simulink model "Cularis_server_vortextest"  (Simulink 8.6)
settings: Solver=FixedStepAuto  SolverMode=SingleTasking  StartTime=0.0  StopTime=uavsim.simConfig.tsim  FixedStep=uavsim.simConfig.tsample_model  RelTol=1
model workspace (MAT data in the model file):
  VortexSig = Simulink.Signal
  VortexSig.DataType = 'Bus: VortexStates'
  VortexSig.Units = 'auto'
  VortexSig.Dimensions = [10 1]
  VortexSig.DimensionsMode = 'Fixed'
  VortexSig.Complexity = 'real'
  VortexSig.SampleTime = -1
  VortexSig.SamplingMode = 'auto'
  VortexSig.InitialValue = 'VortexStates_MATLABStruct_array'
undefined symbols (not defined in the file or in its folder): DiscIntNeverNeededParam, uavsim
libraries: aerolibtransform2 x7, aerolibutil x3, uavsimBlockset_UAV3DInterface x3, uavsimblockset x2, simulink_extras x1, uavsimBlockset_Cularis_withUAV3D x1, aerolibanimutils x1
settings Model: Creator=mstolle  LastModifiedBy=j.bolting  ExtModeTrigDuration=100
settings SolverCC: ZcThreshold=1e-5  ZeroCrossAlgorithm=Adaptive  AlgebraicLoopSolver=LineSearch  AutoInsertRateTranBlk=on
settings DataIOCC: LimitDataPoints=off  SaveFinalState=on  SaveFormat=StructureWithTime  SignalLoggingSaveFormat=Dataset  SaveOutput=off  SaveState=on  DSMLogging=off  InspectSignalLogs=on  StateSaveName=tmp_raccel_xout
settings OptimizationCC: BlockReduction=off  OptimizeBlockIOStorage=off  BufferReuse=off  GlobalBufferReuse=off  ExpressionFolding=off  LocalBlockOutputs=off  EfficientMapNaN2IntZero=off  SimCompilerOptimization=on
settings DebuggingCC: UnderspecifiedInitializationDetection=Simplified  MergeDetectMultiDrivingBlocksExec=error  IgnoredZcDiagnostic=none  FcnCallInpInsideContextMsg=EnableAllAsError  BusObjectLabelMismatch=error
settings HardwareCC: TargetBitPerPointer=64  TargetLongLongMode=on  TargetIntDivRoundTo=Zero  TargetEndianess=LittleEndian  TargetWordSize=64  TargetHWDeviceType=MATLAB Host  ProdEqTarget=off
settings ModelReferenceCC: UpdateModelReferenceTargets=IfOutOfDate  ModelReferenceNumInstancesAllowed=Single  ModelReferenceMinAlgLoopOccurrences=on
settings SFSimCC: SFSimEcho=off
settings RTWCC: SystemTargetFile=raccel.tlc  TemplateMakefile=raccel_default_tmf  RTWVerbose=off  RTWUseSimCustomCode=on
settings CodeAppCC: GenerateComments=off  MaxIdLength=128  SimulinkBlockComments=off
settings RaccelTargetCC: ERTMultiwordTypeDef=System defined  ERTMultiwordLength=256  GeneratePreprocessorConditionals=Use local settings  ERTFirstTimeCompliant=off  MultiInstanceERTCode=off  ENABLE_SLEXEC_SSBRIDGE=0  RTWCAPIParams=on
settings ConfigComp: CovSFcnEnable=off
settings ConfigurationSet: Description=SimMechanics 2G

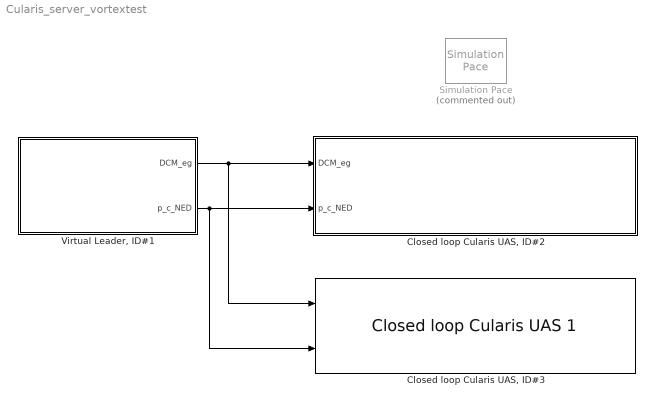
== system Cularis_server_vortextest ==
  "Closed loop Cularis UAS, ID#2" : Subsystem  AncestorBlock=uavsimblockset/Closed loop Cularis UAS 1  mask{closedloopmask_ID=2}
      mask prompts: closedloopmask_ID "UAS ID"
  "Closed loop Cularis UAS, ID#3" : uavsimblockset/Closed loop Cularis UAS 1  closedloopmask_ID=3
  Simulation Pace : aerolibanimutils/Simulation Pace  Commented=on  SimulationPace=1  SleepMode=MATLAB Thread  OutputPaceError=off  SampleTime=-1
  "Virtual Leader, ID#1" : Subsystem  mask{aircraftmask_phithetapsi0=uavsim.formation(1).phithetapsi0, aircraftmask_p0_NED_m=uavsim.formation(1).p0_NED', aircraftmask_originNED_ECEF_rrm=uavsim.originNED_ECEF_radradm, aircraftmask_pqr0=uavsim.formation(1).omega0, aircraftmask_uvw0=uavsim.formation(1).uvw0, aircraftmask_phithetapsi_trim=uavsim.formation(1).phithetapsi0, aircraftmask_ID=1, aircraftmask_wakevortexenabled=on, aircraftmask_navigationLaw=-1, uavsim=uavsim, leaderID=0, airkraftmask_displayLeader=on}
      mask prompts: aircraftmask_phithetapsi0 "Initial Euler angles [rad]"; aircraftmask_p0_NED_m "Initial position, NED frame [m]"; aircraftmask_originNED_ECEF_rrm "Origin NED frame. ECEF, [rad rad m]"; aircraftmask_pqr0 "Initial rotation rates, body frame [rad/s]"; aircraftmask_uvw0 "Initial velocity, body frame [m/s]"; aircraftmask_phithetapsi_trim "Trim Euler angles [rad]"; aircraftmask_ID "Aircraft ID"; aircraftmask_wakevortexenabled "Wake vortex interaction enabled"; aircraftmask_navigationLaw "Active navigation law (-1: automatic selection)"; uavsim "Parameter set"; leaderID "Follows which ID?"; airkraftmask_displayLeader "Display virtual leader"
      mask Display:
      | % Set Icon:
      | %image(imread('images/cularis.png'), [.2, .2, .6, .6])
  wires:
  "Virtual Leader, ID#1"/1(DCM_eg) -> "Closed loop Cularis UAS, ID#2"/1(DCM_eg), "Closed loop Cularis UAS, ID#3"/1
  "Virtual Leader, ID#1"/2(p_c_NED) -> "Closed loop Cularis UAS, ID#2"/2(p_c_NED), "Closed loop Cularis UAS, ID#3"/2

== system Cularis_server_vortextest/Closed loop Cularis UAS, ID#2 ==
  DCM_eg : Inport
  p_c_NED : Inport  Port=2
  Controllers : Subsystem
  UAV : uavsimBlockset_Cularis_withUAV3D/UAV A  aircraftmask_phithetapsi0=uavsim.formation(closedloopmask_ID).phithetapsi0  aircraftmask_p0_NED_m=uavsim.formation(closedloopmask_ID).p0_NED'  aircraftmask_originNED_ECEF_rrm=uavsim.originNED_ECEF_radradm  aircraftmask_pqr0=uavsim.formation(closedloopmask_ID).omega0  aircraftmask_uvw0=uavsim.formation(closedloopmask_ID).uvw0  aircraftmask_phithetapsi_trim=uavsim.formation(closedloopmask_ID).phithetapsi0  aircraftmask_ID=closedloopmask_ID  aircraftmask_wakevortexenabled=off  aircraftmask_navigationLaw=-1  uavsim=uavsim  leaderID=0  aircraftmask_displayUAV3D=on  aircraftmask_displayVortices=off
  wires:
  UAV/1 -> Controllers/1(AirframeBus)
  UAV/2 -> Controllers/2(id)
  DCM_eg/1 -> Controllers/3(DCM_eg)
  p_c_NED/1 -> Controllers/4(p_c_NED)
  Controllers/1(u) -> UAV/1  "u_c"

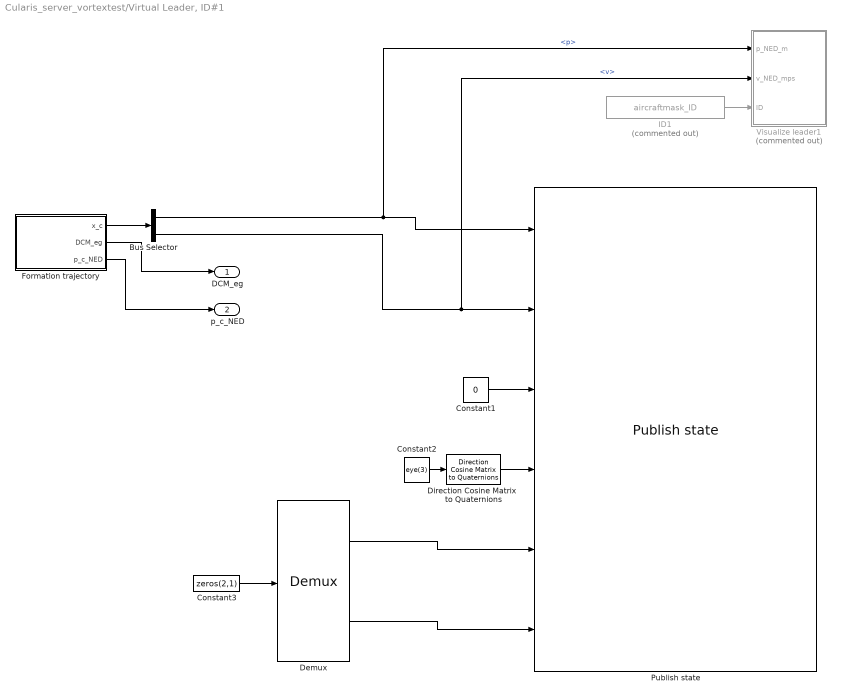
== system Cularis_server_vortextest/Virtual Leader, ID#1 ==
  Bus Selector : BusSelector  OutputSignals=p,v
  Constant1 : Constant  Value=0
  Constant2 : Constant  Value=eye(3)
  Constant3 : Constant  Value=zeros(2,1)
  Demux : Demux  Outputs=2
  Direction Cosine Matrix  to Quaternions : aerolibtransform2/Direction Cosine Matrix  to Quaternions
  Formation trajectory : Subsystem
  ID1 : Constant  Commented=on  Value=aircraftmask_ID
  Publish state : uavsimblockset/Publish state  mask_ID=aircraftmask_ID
  Visualize leader1 : Subsystem  Commented=on  AncestorBlock=formationFlyingBlockset/Visualize leader  TreatAsAtomicUnit=on  SystemSampleTime=uavsim.simConfig.tsample_UAV3D  mask{mask_3dmodel=1}
      mask prompts: mask_3dmodel "3D model"
      mask TypeOptions mask_3dmodel: 0 | 1 | 2 | 3
  DCM_eg : Outport
  p_c_NED : Outport  Port=2
  wires:
  Constant1/1 -> Publish state/3
  Bus Selector/1 -> Publish state/1, Visualize leader1/1(p_NED_m)  "<p>"
  Bus Selector/2 -> Publish state/2, Visualize leader1/2(v_NED_mps)  "<v>"
  Direction Cosine Matrix  to Quaternions/1 -> Publish state/4
  Demux/2 -> Publish state/6
  Demux/1 -> Publish state/5
  Constant2/1 -> Direction Cosine Matrix  to Quaternions/1
  Constant3/1 -> Demux/1
  ID1/1 -> Visualize leader1/3(ID)
  Formation trajectory/1(x_c) -> Bus Selector/1
  Formation trajectory/2(DCM_eg) -> DCM_eg/1
  Formation trajectory/3(p_c_NED) -> p_c_NED/1

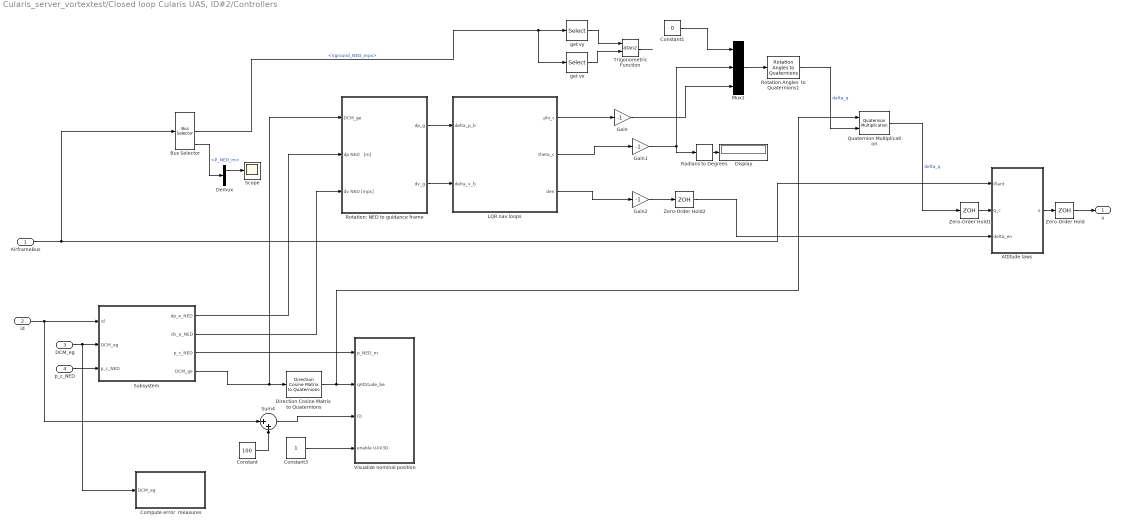
== system Cularis_server_vortextest/Closed loop Cularis UAS, ID#2/Controllers ==
  AirframeBus : Inport
  id : Inport  Port=2
  DCM_eg : Inport  Port=3
  p_c_NED : Inport  Port=4
  Attitude laws : Subsystem  SystemSampleTime=uavsim.ap.hardware.dt_attitudeloops_s
  Bus Selector : BusSelector  OutputSignals=Kinematics.Attitude.DCM_be,Kinematics.Velocity.Vground_NED_mps,Kinematics.Position.P_NED_m
  Compute error  measures : Subsystem
  Constant : Constant  Value=100
  Constant1 : Constant  Value=0
  Constant3 : Constant
  Demux : Demux  Outputs=[2 1]
  Direction Cosine Matrix  to Quaternions : aerolibtransform2/Direction Cosine Matrix  to Quaternions
  Display : Display
  Gain : Gain  Gain=-1
  Gain1 : Gain  Gain=-1
  Gain2 : Gain  Gain=-1
  LQR nav loops : Subsystem  SystemSampleTime=uavsim.ap.hardware.dt_navigationloops_s
  Mux1 : Mux  Inputs=3
  Quaternion Multiplication : aerolibutil/Quaternion Multiplication
  Radians to Degrees : simulink_extras/Transformations/Radians to Degrees
  Rotation Angles  to Quaternions1 : aerolibtransform2/Rotation Angles to Quaternions  rotationOrder=ZYX
  Rotation: NED to guidance frame : Subsystem
  Scope : Scope
  Subsystem : Subsystem
  Sum4 : Sum  Inputs=|++
  Trigonometric Function : Trigonometry  Operator=atan2
  Visualize nominal position : Subsystem  TreatAsAtomicUnit=on  SystemSampleTime=uavsim.simConfig.tsample_UAV3D  mask{mask_3dmodel=1}
      mask prompts: mask_3dmodel "3D model"
      mask TypeOptions mask_3dmodel: 0 | 1 | 2 | 3
  Zero-Order Hold : ZeroOrderHold  SampleTime=uavsim.ap.tsampling_attitudelaws
  Zero-Order Hold1 : ZeroOrderHold  SampleTime=uavsim.ap.tsampling_guidancelaws
  Zero-Order Hold2 : ZeroOrderHold  SampleTime=uavsim.ap.tsampling_guidancelaws
  get vx : Selector  InputPortWidth=3  IndexOptions=Index vector (dialog)  Indices=[1]  OutputSizes=1
  get vy : Selector  InputPortWidth=3  IndexOptions=Index vector (dialog)  Indices=2  OutputSizes=1
  u : Outport
  wires:
  LQR nav loops/3(den) -> Gain2/1
  LQR nav loops/2(theta_c) -> Gain1/1
  LQR nav loops/1(phi_c) -> Gain/1
  Zero-Order Hold/1 -> u/1
  Gain1/1 -> Radians to Degrees/1, Mux1/2
  Trigonometric Function/1 -> ?
  Gain/1 -> Mux1/3
  Mux1/1 -> Rotation Angles  to Quaternions1/1
  get vx/1 -> Trigonometric Function/2
  AirframeBus/1 -> Attitude laws/1(Plant), Bus Selector/1
  get vy/1 -> Trigonometric Function/1
  Attitude laws/1(u) -> Zero-Order Hold/1
  Quaternion Multiplication/1 -> Zero-Order Hold1/1  "delta_q"
  Rotation: NED to guidance frame/2(dv_g) -> LQR nav loops/2(delta_v_b)
  Gain2/1 -> Zero-Order Hold2/1
  Rotation: NED to guidance frame/1(dp_g) -> LQR nav loops/1(delta_p_b)
  Radians to Degrees/1 -> Display/1
  Bus Selector/2 -> get vx/1, get vy/1  "<Vground_NED_mps>"
  Direction Cosine Matrix  to Quaternions/1 -> Quaternion Multiplication/1, Visualize nominal position/2(qAttitude_be)
  Sum4/1 -> Visualize nominal position/3(ID)
  Constant/1 -> Sum4/2
  Constant3/1 -> Visualize nominal position/4(enable UAV3D)
  Zero-Order Hold1/1 -> Attitude laws/2(q_c)
  Zero-Order Hold2/1 -> Attitude laws/3(delta_en)
  id/1 -> Sum4/1, Subsystem/1(id)
  p_c_NED/1 -> Subsystem/3(p_c_NED)
  Subsystem/3("p_c_NED ") -> Visualize nominal position/1(p_NED_m)
  Subsystem/4(DCM_ge) -> Rotation: NED to guidance frame/1(DCM_ge), Direction Cosine Matrix  to Quaternions/1
  Subsystem/1(dp_e_NED) -> Rotation: NED to guidance frame/2(dp NED   [m])
  Subsystem/2(dv_e_NED) -> Rotation: NED to guidance frame/3(dv NED [mps])
  Bus Selector/3 -> Demux/1  "<P_NED_m>"
  Demux/1 -> Scope/1
  DCM_eg/1 -> Compute error  measures/1(DCM_eg), Subsystem/2(DCM_eg)
  Constant1/1 -> Mux1/1
  Rotation Angles  to Quaternions1/1 -> Quaternion Multiplication/2  "delta_q"

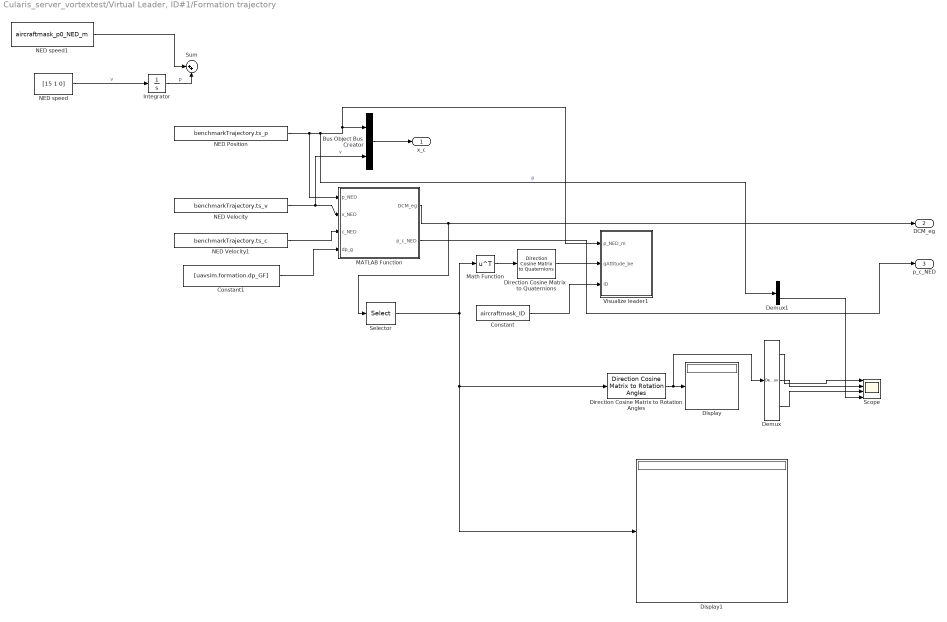
== system Cularis_server_vortextest/Virtual Leader, ID#1/Formation trajectory ==
  Bus Object Bus Creator : BusCreator  Inputs=2  OutDataTypeStr=Bus: svm_bus_x  mask(BUS OBJECT Bus Creator){busType=Bus: svm_bus_x}
      mask prompts: busType "Bus Type"
      mask help:
      | Provides users the cabability to painlessly, instantly customize bus creators of output data type 'Bus:' by selecting the bus object type from a drop down menu dynamically populated by bus objects in the workspace.
      |
      | After pressing the "Apply Selection" button signal lines into the creator are populated and named with the elements in the chosen bus saving the user from having to recall and fill out signal line names.
      |
      | NOTE that when copying a Bus Object Bus Creator from your locked Library the link to the Library is automatically broken. This saves the user from having to Unlock Links To Library (From the Library menu.), Disable Link and finally Break Link (Both from the Model menu.) for every placed instance of the block.
      settings: AttributesFormatString=%<OutDataTypeStr>  CopyFcn=set_param(gcb, 'LinkStatus', 'none')
      mask TypeOptions busType: Bus: AHRS | Bus: Acceleration | Bus: Aero | Bus: Airdata | Bus: Airframe | Bus: Attitude | Bus: CMD | Bus: ControlInfoBus | Bus: Dx | Bus: Enginedata | Bus: Environment | Bus: FlightGearData | Bus: GCSUpstream | Bus: GNSSL1 | Bus: GNSSRTK | Bus: GPS | Bus: IMU | Bus: Kinematics | Bus: LandinggearInput | Bus: MotionTracker | Bus: Position | Bus: Radiodistance | Bus: RotationalAcceleration | Bus: RotationalVelocity | Bus: SensorBus | Bus: StateBus | Bus: Velocity | Bus: VortexParameterBus | Bus: VortexStates | Bus: WindAngles | Bus: iUAScom | Bus: svm_bus_d_exo | Bus: svm_bus_u | Bus: svm_bus_x | Bus: svm_bus_xi
      mask Callback busType:
      | % Using variable names terminated with "_BOBC" to lessen the chances of
      | % collisions with existing workspace variables.
      | 
      | % Get the current block handle and mask handle.
      | handleCreator_BOBC = gcbh;
      | maskObj_BOBC       = Simulink.Mask.get(gcb);
      | 
      | % Get a list of variables in the workspace in order to search for the '1x1
      | % Bus' types.
      | wsVars_BOBC = whos;
      | 
      | % Reset the 'TypeOptions' bus list in case some '1x1 Bus' types have been
      | % deleted from or added to the workspace.
      | maskObj_BOBC.Parameters.TypeOptions = {'<empty>'};
      | 
      | % Reset the bus count.
      | busCount_BOBC = 0;
      | 
      | for index_BOBC = 1:length(wsVars_BOBC)
      | 
      |    % If the variable is a bus object...
      |    if strcmp(wsVars_BOBC(index_BOBC).class, 'Simulink.Bus')
      | 
      |       busCount_BOBC = busCount_BOBC + 1;
      | 
      |       % ... add it to the TypeOptions of the mask.
      |       maskObj_BOBC.Parameters.TypeOptions(busCount_BOBC) = ...
      |                                                            ...
      |                                  {['Bus: ', wsVars_BOBC(index_BOBC).name]};
      |    end
      | end
      | 
      | if busCount_BOBC == 0
      | 
      |    % If there are NO bus objects in the workspace then provide a warning
      |    % popup...
      |    warndlg('There are currently no bus objects in the workspace - you have no use for this block. Use a normal Bus Creator instead.')
      | 
      |    % ... and do nothing.
      | elseif ~strcmp(get_param(handleCreator_BOBC, 'OutDataTypeStr'), 'Inherit: auto')
      | 
      |    % If the currently selected bus data type ('OutDataTypeStr') is not
      |    % 'Inherit: auto' (i.e., if we are reopening the mask.) then get the
      |    % current 'OutDataTypeStr' and 'maskVal.' ('maskVal' is the selected
      |    % 'TypeOptions' list member.)
      |    outDatStr_BOBC = get_param(handleCreator_BOBC, 'OutDataTypeStr');
      |    maskVal_BOBC   = get_param(handleCreator_BOBC, 'MaskValues');
      | 
      |    if ~strcmp(outDatStr_BOBC, maskVal_BOBC{1})
      | 
      |       % Upon re-opening the mask if the default 'TypeOptions' list member
      |       % (The first one.) contained in 'maskVal' does not match the
      |       % currently selected bus data type ('OutDataTypeStr') then set the
      |       % 'TypeOptions' list member to the selected bus data type. (Cuts down
      |       % on confusion to have the displayed list member match the selected
      |       % bus data type rather than the first entry.)
      |       set_param(handleCreator_BOBC, 'MaskValues', {outDatStr_BOBC});
      |    end
      | end
      | 
      | % Clean up the workspace.
      | clear  handleCreator_BOBC  maskObj_BOBC     wsVars_BOBC ...
      |             busCount_BOBC    index_BOBC  outDatStr_BOBC ...
      |              maskVal_BOBC
      mask DialogControl applyMOCBSelection Prompt: Apply Selection
      mask DialogControl applyMOCBSelection Callback:
      | % Using variable names terminated with "_BOBC" to lessen the chances of
      | % collisions with existing workspace variables.
      | 
      | % Get the current block, current block handle and mask handle.
      | currentBlock_BOBC  = gcb;
      | handleCreator_BOBC = gcbh;
      | 
      | % Get the desired bus type...
      | desiredBusType_BOBC = get_param(handleCreator_BOBC, 'busType');
      | 
      | % ... and set the 'OutDataTypeStr' to it.
      | set_param(handleCreator_BOBC, 'OutDataTypeStr', desiredBusType_BOBC);
      | 
      | %% First delete any existing lines on the port.
      | % Get the line handles.
      | lh_BOBC = get_param(handleCreator_BOBC, 'LineHandles');
      | 
      | % If any lines exist (Non- -1 line handles.), delete them and start over.
      | if max(lh_BOBC.Inport > 0)
      | 
      |    for index_BOBC = 1:length(lh_BOBC.Inport)
      | 
      |       if lh_BOBC.Inport(index_BOBC) > 0
      | 
      |          delete_line(lh_BOBC.Inport(index_BOBC))
      |       end
      |    end
      | end
      | 
      | %% Then work on adding new lines.
      | 
      | % Get the block path for 'add_line' function.
      | blockPath_BOBC = get_param(handleCreator_BOBC, 'Parent');
      | 
      | % Get the newly selected bus type ('OutDataTypeStr')...
      | mocbBusType_BOBC = get_param(currentBlock_BOBC, 'OutDataTypeStr');
      | 
      | % ... and parse off "Bus: " so the string of the desired bus contained in
      | % 'OutDataTypeStr' matches the raw workspace bus names.
      | mocbBusType_BOBC = mocbBusType_BOBC(6:end);
      | 
      | % Then evaluate the string containing the workspace bus name which will
      | % load the desired bus parameters.
      | busParams_BOBC = eval(mocbBusType_BOBC);
      | 
      | % From the parameters grab the number of lines to add.
      | numLines_BOBC = length(busParams_BOBC.Elements);
      | 
      | % Set the number of inputs of the masked bus creator to the number of lines
      | % to add.
      | set_param(handleCreator_BOBC, 'Inputs', num2str(numLines_BOBC));
      | 
      | % Get (Inputs.) port handles so we can grab the positions of them.
      | ph_BOBC = get_param(handleCreator_BOBC, 'PortHandles');
      | 
      | for index_BOBC = 1:numLines_BOBC
      | 
      |    % Get the position of input port number 'index_BOBC'.
      |    portPos_BOBC = get_param(ph_BOBC.Inport(index_BOBC), 'Position');
      | 
      |    % Add a line from 50 pixels left of the port position to the port
      |    % position. (This must be done because it's the lines that get named,
      |    % not the port positions.)
      |    portLine_BOBC = add_line(blockPath_BOBC, [portPos_BOBC - [50 0]; portPos_BOBC]);
      | 
      |    % Rename the new line to the bus 'index_BOBC-st/nd/rd/th' element name.
      |    set_param(portLine_BOBC, 'Name', busParams_BOBC.Elements(index_BOBC).Name)
      | end
      | 
      | %% Cleanup the workspace.
      | clear    currentBlock_BOBC  handleCreator_BOBC      index_BOBC ...
      |        desiredBusType_BOBC             lh_BOBC  blockPath_BOBC ...
      |           mocbBusType_BOBC      busParams_BOBC   numLines_BOBC ...
      |                    ph_BOBC        portPos_BOBC   portLine_BOBC
  Constant : Constant  Value=aircraftmask_ID
  Constant1 : Constant  Value=[uavsim.formation.dp_GF]
  Demux : Demux  Outputs=3
  Demux1 : Demux  Outputs=3
  Direction Cosine Matrix to Rotation Angles : aerolibtransform2/Direction Cosine Matrix to Rotation Angles  rotationOrder=ZYX  lim=Default
      settings: AttributesFormatString=Rotation Order: %<rotationOrder>
  Direction Cosine Matrix  to Quaternions : aerolibtransform2/Direction Cosine Matrix  to Quaternions
  Display : Display
      settings: Decimation=3
  Display1 : Display
      settings: Decimation=3
  Integrator : Integrator  InitialCondition=[0 0 0]
  MATLAB Function : MATLAB Function  TreatAsAtomicUnit=on
  Math Function : Math  Operator=transpose  SaturateOnIntegerOverflow=on
  NED Position : FromWorkspace  VariableName=benchmarkTrajectory.ts_p  SampleTime=0
  NED Velocity : FromWorkspace  VariableName=benchmarkTrajectory.ts_v  SampleTime=0
  NED Velocity1 : FromWorkspace  VariableName=benchmarkTrajectory.ts_c  SampleTime=0
  NED speed : Constant  Value=[15 1 0]
  NED speed1 : Constant  Value=aircraftmask_p0_NED_m
  Scope : Scope  NumInputPorts=4
  Selector : Selector  NumberOfDimensions=3  InputPortWidth=3  IndexOptions=Index vector (dialog),Index vector (dialog),Index vector (dialog)  Indices=1:3,1:3,1  OutputSizes=1,1,1
  Sum : Sum  Inputs=|++
  Visualize leader1 : Subsystem  TreatAsAtomicUnit=on  SystemSampleTime=uavsim.simConfig.tsample_UAV3D  mask{mask_3dmodel=3}
      mask prompts: mask_3dmodel "3D model"
      mask TypeOptions mask_3dmodel: 0 | 1 | 2 | 3
  x_c : Outport  OutDataTypeStr=Bus: svm_bus_x
  DCM_eg : Outport  Port=2
  p_c_NED : Outport  Port=3
  wires:
  NED Position/1 -> MATLAB Function/1(p_NED), Demux1/1, Visualize leader1/1(p_NED_m), Bus Object Bus Creator/1  "p"
  NED speed/1 -> Integrator/1  "v"
  Bus Object Bus Creator/1 -> x_c/1
  Integrator/1 -> Sum/2  "p"
  NED speed1/1 -> Sum/1
  NED Velocity/1 -> MATLAB Function/2(v_NED), Bus Object Bus Creator/2  "v"
  NED Velocity1/1 -> MATLAB Function/3(c_NED)
  Selector/1 -> Display1/1, Direction Cosine Matrix to Rotation Angles/1, Math Function/1
  Direction Cosine Matrix  to Quaternions/1 -> Visualize leader1/2(qAttitude_be)
  Constant/1 -> Visualize leader1/3(ID)
  Direction Cosine Matrix to Rotation Angles/1 -> Demux/1, Display/1
  Demux/2 -> Scope/2
  Demux/3 -> Scope/3
  Demux/1 -> Scope/1
  Demux1/3 -> Scope/4
  Constant1/1 -> MATLAB Function/4(dp_g)
  MATLAB Function/1(DCM_eg) -> Selector/1, DCM_eg/1
  MATLAB Function/2(p_c_NED) -> p_c_NED/1
  Math Function/1 -> Direction Cosine Matrix  to Quaternions/1

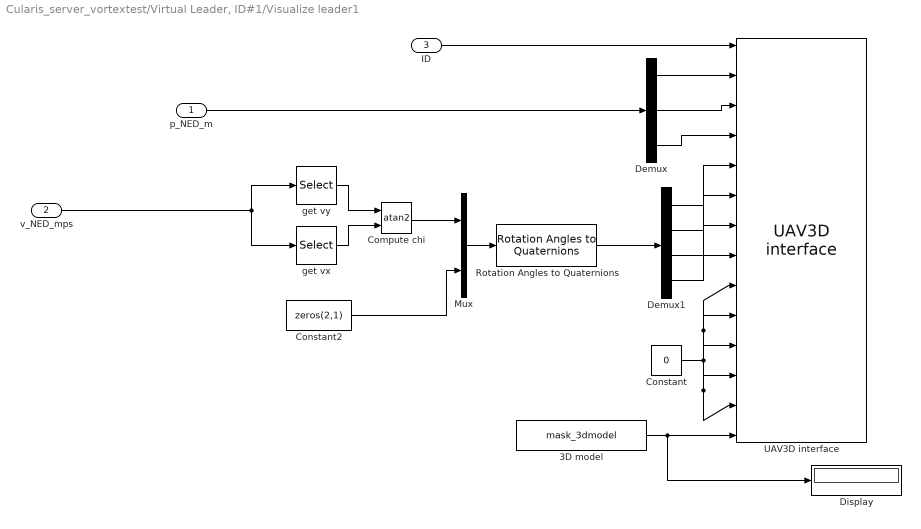
== system Cularis_server_vortextest/Virtual Leader, ID#1/Visualize leader1 ==
  p_NED_m : Inport
  v_NED_mps : Inport  Port=2
  ID : Inport  Port=3
  3D model : Constant  Value=mask_3dmodel
  Compute chi : Trigonometry  Operator=atan2
  Constant : Constant  Value=0
  Constant2 : Constant  Value=zeros(2,1)
  Demux : Demux  Outputs=3
  Demux1 : Demux
  Display : Display
  Mux : Mux  Inputs=2
  Rotation Angles to Quaternions : aerolibtransform2/Rotation Angles to Quaternions  rotationOrder=ZYX
  UAV3D interface : uavsimBlockset_UAV3DInterface/UAV3D interface  ip='localhost'  udpport=4445
  get vx : Selector  InputPortWidth=3  IndexOptions=Index vector (dialog)  Indices=1  OutputSizes=1
  get vy : Selector  InputPortWidth=3  IndexOptions=Index vector (dialog)  Indices=2  OutputSizes=1
  wires:
  Demux/1 -> UAV3D interface/2
  Demux/2 -> UAV3D interface/3
  Demux/3 -> UAV3D interface/4
  Demux1/1 -> UAV3D interface/5
  Demux1/2 -> UAV3D interface/6
  Demux1/4 -> UAV3D interface/8
  get vy/1 -> Compute chi/1
  get vx/1 -> Compute chi/2
  Constant2/1 -> Mux/2
  Mux/1 -> Rotation Angles to Quaternions/1
  Rotation Angles to Quaternions/1 -> Demux1/1
  Compute chi/1 -> Mux/1
  Demux1/3 -> UAV3D interface/7
  Constant/1 -> UAV3D interface/13, UAV3D interface/12, UAV3D interface/11, UAV3D interface/10, UAV3D interface/9
  3D model/1 -> Display/1, UAV3D interface/14
  ID/1 -> UAV3D interface/1
  p_NED_m/1 -> Demux/1
  v_NED_mps/1 -> get vy/1, get vx/1

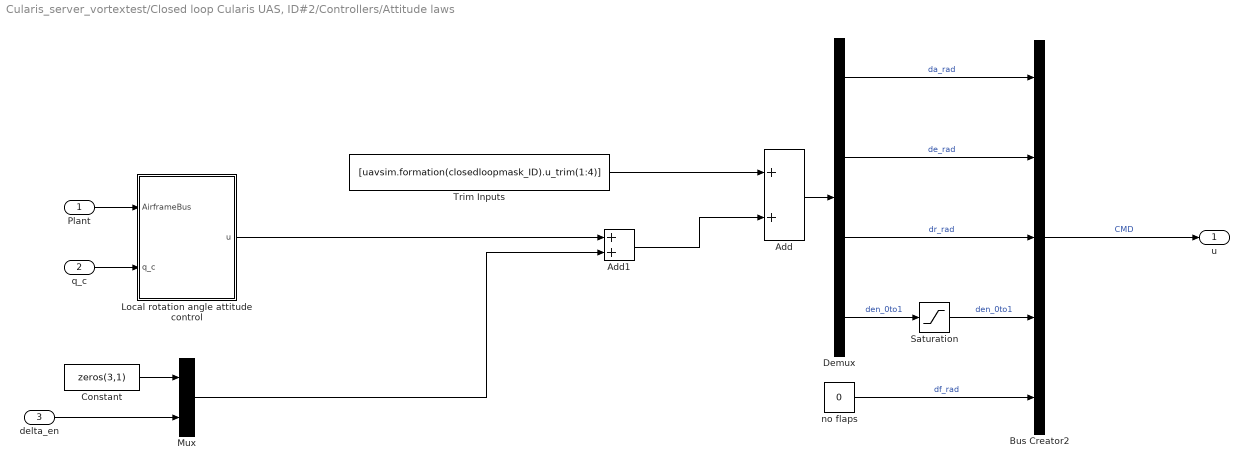
== system Cularis_server_vortextest/Closed loop Cularis UAS, ID#2/Controllers/Attitude laws ==
  Plant : Inport  OutDataTypeStr=Bus: Airframe
  q_c : Inport  Port=2
  delta_en : Inport  Port=3
  Add : Sum
  Add1 : Sum
  Bus Creator2 : BusCreator  Inputs=5  OutDataTypeStr=Bus: CMD  NonVirtualBus=on
  Constant : Constant  Value=zeros(3,1)
  Demux : Demux
  Local rotation angle attitude  control : Subsystem
  Mux : Mux  Inputs=2
  Saturation : Saturate  UpperLimit=1  LowerLimit=0
  Trim Inputs : Constant  Value=[uavsim.formation(closedloopmask_ID).u_trim(1:4)]
  no flaps : Constant  Value=0
  u : Outport  OutDataTypeStr=Bus: CMD
  wires:
  no flaps/1 -> Bus Creator2/5  "df_rad"
  delta_en/1 -> Mux/2
  Add1/1 -> Add/2
  Mux/1 -> Add1/2
  Constant/1 -> Mux/1
  q_c/1 -> Local rotation angle attitude  control/2(q_c)
  Plant/1 -> Local rotation angle attitude  control/1(AirframeBus)
  Add/1 -> Demux/1
  Trim Inputs/1 -> Add/1
  Demux/2 -> Bus Creator2/2  "de_rad"
  Demux/1 -> Bus Creator2/1  "da_rad"
  Saturation/1 -> Bus Creator2/4  "den_0to1"
  Demux/3 -> Bus Creator2/3  "dr_rad"
  Bus Creator2/1 -> u/1  "CMD"
  Local rotation angle attitude  control/1(u) -> Add1/1
  Demux/4 -> Saturation/1  "den_0to1"

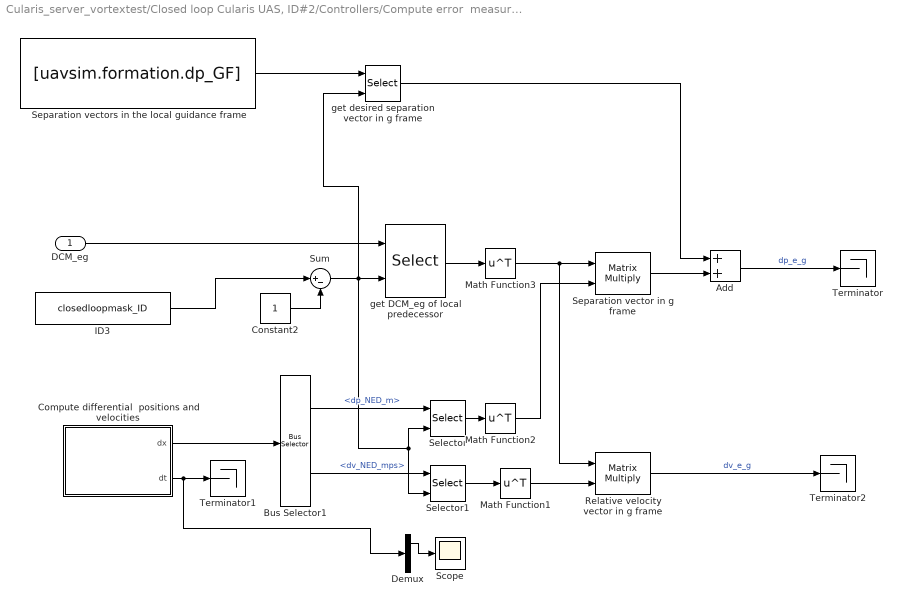
== system Cularis_server_vortextest/Closed loop Cularis UAS, ID#2/Controllers/Compute error  measures ==
  DCM_eg : Inport
  Add : Sum
  Bus Selector1 : BusSelector  OutputSignals=dp_NED_m,dv_NED_mps
  Compute differential  positions and velocities : MATLAB Function  TreatAsAtomicUnit=on
  Constant2 : Constant
  Demux : Demux  Outputs=[4 6]
  ID3 : Constant  Value=closedloopmask_ID
  Math Function1 : Math  Operator=transpose  SaturateOnIntegerOverflow=on
  Math Function2 : Math  Operator=transpose  SaturateOnIntegerOverflow=on
  Math Function3 : Math  Operator=transpose  SaturateOnIntegerOverflow=on
  Relative velocity vector in g frame : Product  Multiplication=Matrix(*)
  Scope : Scope
  Selector : Selector  NumberOfDimensions=2  InputPortWidth=3  IndexOptions=Index vector (port),Select all  Indices=1,1:3  OutputSizes=1,1
  Selector1 : Selector  NumberOfDimensions=2  InputPortWidth=3  IndexOptions=Index vector (port),Index vector (dialog)  Indices=1,1:3  OutputSizes=1,1
  Separation vector in g frame : Product  Multiplication=Matrix(*)
  Separation vectors in the local guidance frame : Constant  Value=[uavsim.formation.dp_GF]
  Sum : Sum  Inputs=|+-
  Terminator : Terminator
  Terminator1 : Terminator
  Terminator2 : Terminator
  get DCM_eg of local predecessor : Selector  NumberOfDimensions=3  InputPortWidth=3  IndexOptions=Index vector (dialog),Index vector (dialog),Index vector (port)  Indices=1:3,1:3,1  OutputSizes=1,1,1
  get desired separation vector in g frame : Selector  NumberOfDimensions=2  InputPortWidth=3  IndexOptions=Select all,Index vector (port)  Indices=1,1:3  OutputSizes=1,1
  wires:
  Separation vectors in the local guidance frame/1 -> get desired separation vector in g frame/1
  DCM_eg/1 -> get DCM_eg of local predecessor/1
  Constant2/1 -> Sum/2
  Bus Selector1/1 -> Selector/1  "<dp_NED_m>"
  Bus Selector1/2 -> Selector1/1  "<dv_NED_mps>"
  Compute differential  positions and velocities/1(dx) -> Bus Selector1/1
  Selector/1 -> Math Function2/1
  ID3/1 -> Sum/1
  Sum/1 -> get desired separation vector in g frame/2, Selector1/2, Selector/2, get DCM_eg of local predecessor/2
  get DCM_eg of local predecessor/1 -> Math Function3/1
  Math Function2/1 -> Separation vector in g frame/2
  Selector1/1 -> Math Function1/1
  Separation vector in g frame/1 -> Add/2
  Add/1 -> Terminator/1  "dp_e_g"
  Relative velocity vector in g frame/1 -> Terminator2/1  "dv_e_g"
  Math Function1/1 -> Relative velocity vector in g frame/2
  Math Function3/1 -> Relative velocity vector in g frame/1, Separation vector in g frame/1
  Compute differential  positions and velocities/2(dt) -> Demux/1, Terminator1/1
  get desired separation vector in g frame/1 -> Add/1
  Demux/1 -> Scope/1

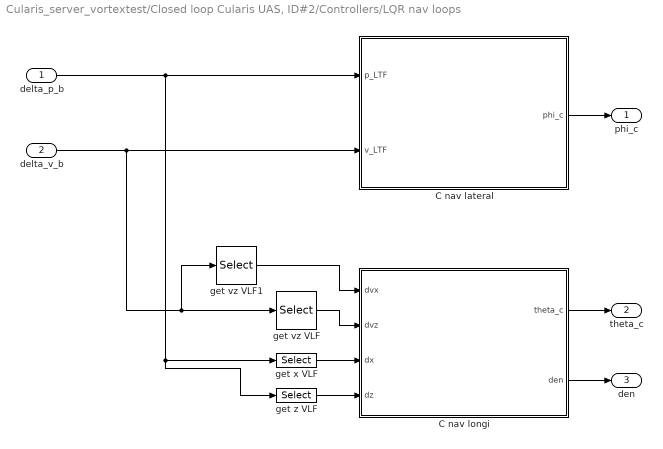
== system Cularis_server_vortextest/Closed loop Cularis UAS, ID#2/Controllers/LQR nav loops ==
  delta_p_b : Inport
  delta_v_b : Inport  Port=2
  C nav lateral : Subsystem
  C nav longi : Subsystem
  get vz VLF : Selector  InputPortWidth=3  IndexOptions=Index vector (dialog)  Indices=3  OutputSizes=1
  get vz VLF1 : Selector  InputPortWidth=3  IndexOptions=Index vector (dialog)  Indices=1  OutputSizes=1
  get x VLF : Selector  InputPortWidth=3  IndexOptions=Index vector (dialog)  Indices=1  OutputSizes=1
  get z VLF : Selector  InputPortWidth=3  IndexOptions=Index vector (dialog)  Indices=3  OutputSizes=1
  phi_c : Outport  PortDimensions=1
  theta_c : Outport  Port=2  PortDimensions=1
  den : Outport  Port=3  PortDimensions=1
  wires:
  C nav longi/2(den) -> den/1
  C nav longi/1(theta_c) -> theta_c/1
  delta_p_b/1 -> C nav lateral/1(p_LTF), get x VLF/1, get z VLF/1
  delta_v_b/1 -> C nav lateral/2(v_LTF), get vz VLF1/1, get vz VLF/1
  C nav lateral/1(phi_c) -> phi_c/1
  get z VLF/1 -> C nav longi/4(dz)
  get x VLF/1 -> C nav longi/3(dx)
  get vz VLF/1 -> C nav longi/2(dvz)
  get vz VLF1/1 -> C nav longi/1(dvx)

== system Cularis_server_vortextest/Closed loop Cularis UAS, ID#2/Controllers/Rotation: NED to guidance frame ==
  DCM_ge : Inport
  dp NED   [m] : Inport  Port=2
  dv NED [mps] : Inport  Port=3
  Rotate position vector from NED to LS frame : Product  Multiplication=Matrix(*)
  Rotate velocity vector from NED to LS frame : Product  Multiplication=Matrix(*)
  dp_g : Outport
  dv_g : Outport  Port=2
  wires:
  Rotate velocity vector from NED to LS frame/1 -> dv_g/1
  Rotate position vector from NED to LS frame/1 -> dp_g/1
  dp NED   [m]/1 -> Rotate position vector from NED to LS frame/2
  dv NED [mps]/1 -> Rotate velocity vector from NED to LS frame/2
  DCM_ge/1 -> Rotate velocity vector from NED to LS frame/1, Rotate position vector from NED to LS frame/1

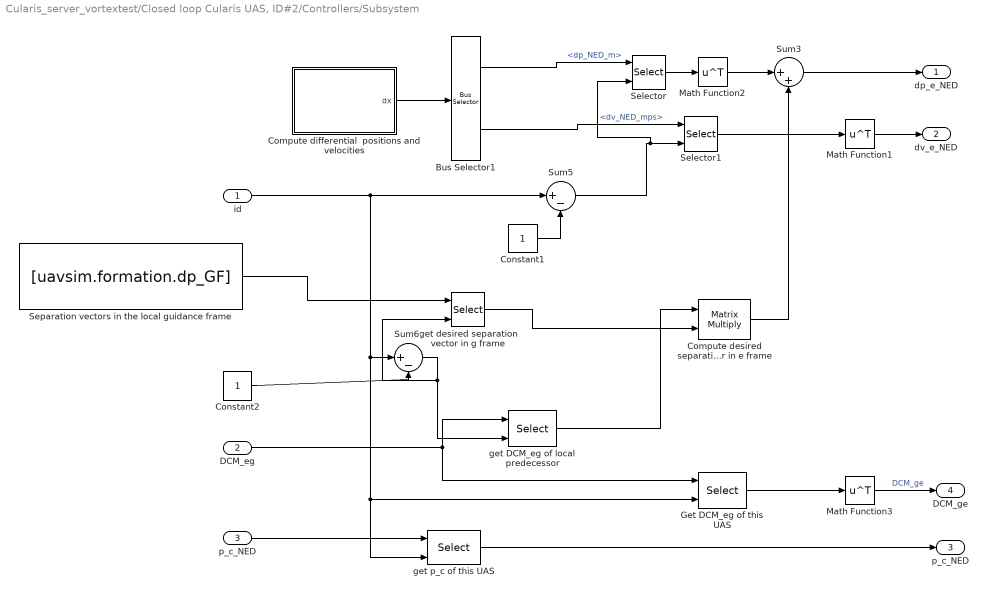
== system Cularis_server_vortextest/Closed loop Cularis UAS, ID#2/Controllers/Subsystem ==
  id : Inport
  DCM_eg : Inport  Port=2
  p_c_NED : Inport  Port=3
  Bus Selector1 : BusSelector  OutputSignals=dp_NED_m,dv_NED_mps
  Compute desired separation vector in e frame : Product  Multiplication=Matrix(*)
  Compute differential  positions and velocities : MATLAB Function  TreatAsAtomicUnit=on
  Constant1 : Constant
  Constant2 : Constant
  Get DCM_eg of this UAS : Selector  NumberOfDimensions=3  InputPortWidth=3  IndexOptions=Index vector (dialog),Index vector (dialog),Index vector (port)  Indices=1:3,1:3,1  OutputSizes=1,1,1
  Math Function1 : Math  Operator=transpose  SaturateOnIntegerOverflow=on
  Math Function2 : Math  Operator=transpose  SaturateOnIntegerOverflow=on
  Math Function3 : Math  Operator=transpose  SaturateOnIntegerOverflow=on
  Selector : Selector  NumberOfDimensions=2  InputPortWidth=3  IndexOptions=Index vector (port),Select all  Indices=1,1:3  OutputSizes=1,1
  Selector1 : Selector  NumberOfDimensions=2  InputPortWidth=3  IndexOptions=Index vector (port),Index vector (dialog)  Indices=1,1:3  OutputSizes=1,1
  Separation vectors in the local guidance frame : Constant  Value=[uavsim.formation.dp_GF]
  Sum3 : Sum  Inputs=|++
  Sum5 : Sum  Inputs=|+-
  Sum6 : Sum  Inputs=|+-
  get DCM_eg of local predecessor : Selector  NumberOfDimensions=3  InputPortWidth=3  IndexOptions=Index vector (dialog),Index vector (dialog),Index vector (port)  Indices=1:3,1:3,1  OutputSizes=1,1,1
  get desired separation vector in g frame : Selector  NumberOfDimensions=2  InputPortWidth=3  IndexOptions=Select all,Index vector (port)  Indices=1,1:3  OutputSizes=1,1
  get p_c of this UAS : Selector  NumberOfDimensions=2  InputPortWidth=3  IndexOptions=Select all,Index vector (port)  Indices=1,1:3  OutputSizes=1,1
  dp_e_NED : Outport
  dv_e_NED : Outport  Port=2
  "p_c_NED " : Outport  Port=3
  DCM_ge : Outport  Port=4
  wires:
  Sum3/1 -> dp_e_NED/1
  Math Function1/1 -> dv_e_NED/1
  p_c_NED/1 -> get p_c of this UAS/1
  get p_c of this UAS/1 -> "p_c_NED "/1
  Constant1/1 -> Sum5/2
  Math Function3/1 -> DCM_ge/1  "DCM_ge"
  Sum5/1 -> Selector/2, Selector1/2
  Compute differential  positions and velocities/1(dx) -> Bus Selector1/1
  Selector1/1 -> Math Function1/1
  Bus Selector1/2 -> Selector1/1  "<dv_NED_mps>"
  Bus Selector1/1 -> Selector/1  "<dp_NED_m>"
  get DCM_eg of local predecessor/1 -> Compute desired separation vector in e frame/1
  Constant2/1 -> Sum6/2
  Sum6/1 -> get DCM_eg of local predecessor/2, get desired separation vector in g frame/2
  Selector/1 -> Math Function2/1
  DCM_eg/1 -> get DCM_eg of local predecessor/1, Get DCM_eg of this UAS/1
  Separation vectors in the local guidance frame/1 -> get desired separation vector in g frame/1
  Get DCM_eg of this UAS/1 -> Math Function3/1
  get desired separation vector in g frame/1 -> Compute desired separation vector in e frame/2
  Math Function2/1 -> Sum3/1
  Compute desired separation vector in e frame/1 -> Sum3/2
  id/1 -> Sum6/1, get p_c of this UAS/2, Get DCM_eg of this UAS/2, Sum5/1

== system Cularis_server_vortextest/Closed loop Cularis UAS, ID#2/Controllers/Visualize nominal position ==
  p_NED_m : Inport
  qAttitude_be : Inport  Port=2
  ID : Inport  Port=3
  enable UAV3D : Inport  Port=4
  3D model : Constant  Value=mask_3dmodel
  Constant : Constant  Value=0
  Demux : Demux  Outputs=3
  Demux1 : Demux
  UAV3D interface : uavsimBlockset_UAV3DInterface/UAV3D interface  ip='localhost'  udpport=4445
  wires:
  Demux/1 -> UAV3D interface/2
  Demux/2 -> UAV3D interface/3
  Demux/3 -> UAV3D interface/4
  Demux1/1 -> UAV3D interface/5
  Demux1/2 -> UAV3D interface/6
  Demux1/4 -> UAV3D interface/8
  qAttitude_be/1 -> Demux1/1
  Demux1/3 -> UAV3D interface/7
  Constant/1 -> UAV3D interface/13, UAV3D interface/12, UAV3D interface/11, UAV3D interface/10, UAV3D interface/9
  3D model/1 -> UAV3D interface/14
  ID/1 -> UAV3D interface/1
  p_NED_m/1 -> Demux/1
  enable UAV3D/1 -> UAV3D interface/Enable

== system Cularis_server_vortextest/Virtual Leader, ID#1/Formation trajectory/Visualize leader1 ==
  p_NED_m : Inport
  qAttitude_be : Inport  Port=2
  ID : Inport  Port=3
  3D model : Constant  Value=mask_3dmodel
  Constant : Constant  Value=0
  Constant1 : Constant
  Demux : Demux  Outputs=3
  Demux1 : Demux
  UAV3D interface : uavsimBlockset_UAV3DInterface/UAV3D interface  ip='localhost'  udpport=4445
  wires:
  Demux/1 -> UAV3D interface/2
  Demux/2 -> UAV3D interface/3
  Demux/3 -> UAV3D interface/4
  Demux1/1 -> UAV3D interface/5
  Demux1/2 -> UAV3D interface/6
  Demux1/4 -> UAV3D interface/8
  qAttitude_be/1 -> Demux1/1
  Demux1/3 -> UAV3D interface/7
  Constant/1 -> UAV3D interface/13, UAV3D interface/12, UAV3D interface/11, UAV3D interface/10, UAV3D interface/9
  3D model/1 -> UAV3D interface/14
  ID/1 -> UAV3D interface/1
  p_NED_m/1 -> Demux/1
  Constant1/1 -> UAV3D interface/Enable

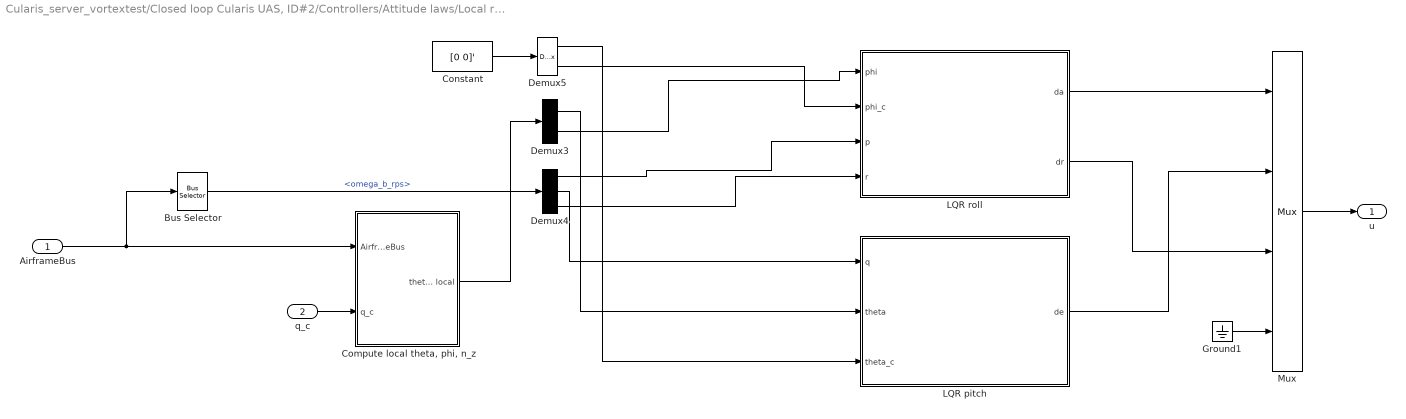
== system Cularis_server_vortextest/Closed loop Cularis UAS, ID#2/Controllers/Attitude laws/Local rotation angle attitude  control ==
  AirframeBus : Inport  OutDataTypeStr=Bus: Airframe
  q_c : Inport  Port=2
  Bus Selector : BusSelector  OutputSignals=Kinematics.RotationalVelocity.omega_b_rps
  "Compute local theta, phi, n_z" : Subsystem
  Constant : Constant  Value=[0 0]'
  Demux3 : Demux  Outputs=2
  Demux4 : Demux  Outputs=3
  Demux5 : Demux  Outputs=2
  Ground1 : Ground
  LQR pitch : Subsystem
  LQR roll : Subsystem
  Mux : Mux
  u : Outport
  wires:
  Ground1/1 -> Mux/4
  AirframeBus/1 -> "Compute local theta, phi, n_z"/1(AirframeBus), Bus Selector/1
  q_c/1 -> "Compute local theta, phi, n_z"/2(q_c)
  Mux/1 -> u/1
  Constant/1 -> Demux5/1
  Bus Selector/1 -> Demux4/1  "<omega_b_rps>"
  "Compute local theta, phi, n_z"/1("theta, phi local") -> Demux3/1
  Demux5/2 -> LQR roll/2(phi_c)
  Demux3/2 -> LQR roll/1(phi)
  Demux4/1 -> LQR roll/3(p)
  Demux4/3 -> LQR roll/4(r)
  Demux5/1 -> LQR pitch/3(theta_c)
  Demux3/1 -> LQR pitch/2(theta)
  Demux4/2 -> LQR pitch/1(q)
  LQR pitch/1(de) -> Mux/2
  LQR roll/1(da) -> Mux/1
  LQR roll/2(dr) -> Mux/3

== system Cularis_server_vortextest/Closed loop Cularis UAS, ID#2/Controllers/LQR nav loops/C nav lateral ==
  p_LTF : Inport
  v_LTF : Inport  Port=2
  Add : Sum  Inputs=+-
  Discrete-Time Integrator1 : DiscreteIntegrator  SampleTime=-1  ICPrevOutput=DiscIntNeverNeededParam  ICPrevScaledInput=DiscIntNeverNeededParam
  Ky : Gain  Gain=uavsim.ap.control.lquadr.latnav.K  Multiplication=Matrix(K*u)
  Mux1 : Mux  Inputs=3
  Selector : Selector  InputPortWidth=3  IndexOptions=Index vector (dialog)  Indices=2  OutputSizes=1
  Selector1 : Selector  InputPortWidth=3  IndexOptions=Index vector (dialog)  Indices=2  OutputSizes=1
  Step : Step  Time=12  After=0
  Trigonometric Function : Trigonometry  Operator=asin
  phi_c : Outport
  wires:
  Ky/1 -> Trigonometric Function/1  "ny_c"
  Selector/1 -> Add/1  "e"
  Step/1 -> Add/2
  Selector1/1 -> Mux1/2
  Discrete-Time Integrator1/1 -> Mux1/3
  Add/1 -> Mux1/1, Discrete-Time Integrator1/1
  Mux1/1 -> Ky/1
  v_LTF/1 -> Selector1/1
  p_LTF/1 -> Selector/1
  Trigonometric Function/1 -> phi_c/1

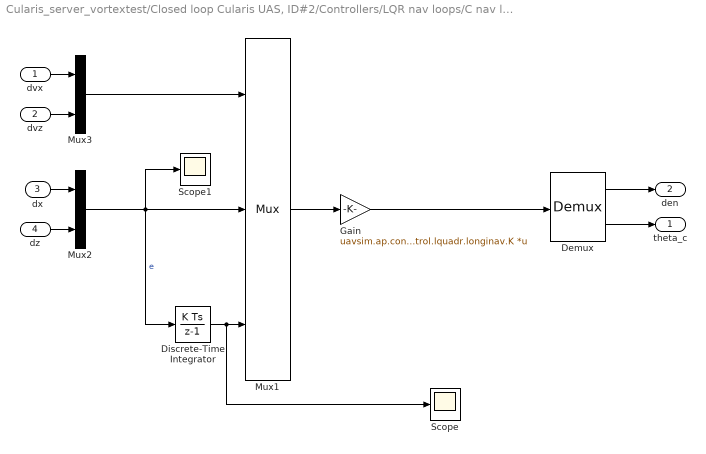
== system Cularis_server_vortextest/Closed loop Cularis UAS, ID#2/Controllers/LQR nav loops/C nav longi ==
  dvx : Inport
  dvz : Inport  Port=2
  dx : Inport  Port=3
  dz : Inport  Port=4
  Demux : Demux  Outputs=2
  Discrete-Time Integrator : DiscreteIntegrator  gainval=1  InitialConditionSetting=State (most efficient)  SampleTime=-1  ICPrevOutput=DiscIntNeverNeededParam  ICPrevScaledInput=DiscIntNeverNeededParam
  Gain : Gain  Gain=uavsim.ap.control.lquadr.longinav.K  Multiplication=Matrix(K*u)
  Mux1 : Mux  Inputs=3
  Mux2 : Mux  Inputs=2
  Mux3 : Mux  Inputs=2
  Scope : Scope
  Scope1 : Scope
  theta_c : Outport
  den : Outport  Port=2
  wires:
  Mux1/1 -> Gain/1
  Demux/1 -> den/1
  Demux/2 -> theta_c/1
  dx/1 -> Mux2/1
  dvz/1 -> Mux3/2
  dvx/1 -> Mux3/1
  Discrete-Time Integrator/1 -> Scope/1, Mux1/3
  Mux2/1 -> Discrete-Time Integrator/1, Scope1/1, Mux1/2  "e"
  Gain/1 -> Demux/1
  dz/1 -> Mux2/2
  Mux3/1 -> Mux1/1

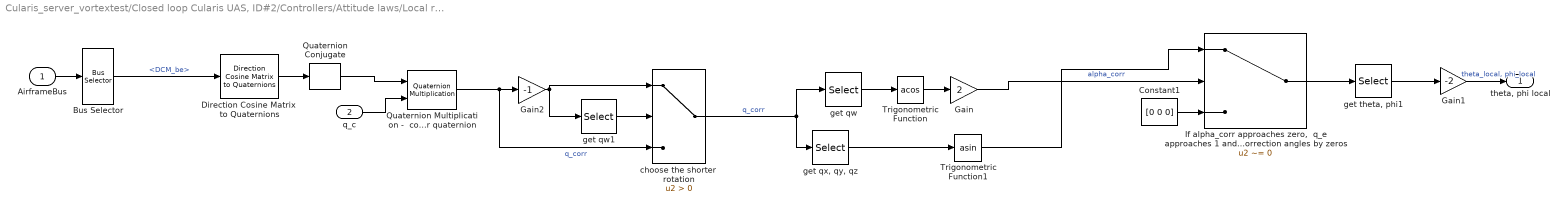
== system Cularis_server_vortextest/Closed loop Cularis UAS, ID#2/Controllers/Attitude laws/Local rotation angle attitude  control/Compute local theta, phi, n_z ==
  AirframeBus : Inport  OutDataTypeStr=Bus: Airframe
  q_c : Inport  Port=2
  Bus Selector : BusSelector  OutputSignals=Kinematics.Attitude.DCM_be
  Constant1 : Constant  Value=[0 0 0]
  Direction Cosine Matrix  to Quaternions : aerolibtransform2/Direction Cosine Matrix  to Quaternions
  Gain : Gain  Gain=2
  Gain1 : Gain  Gain=-2
  Gain2 : Gain  Gain=-1
  "If alpha_corr approaches zero,  q_e approaches 1 and c goes to infinity.  In that case, just replace the computed  correction angles by zeros" : Switch  Criteria=u2 ~= 0
  Quaternion Conjugate : aerolibutil/Quaternion Conjugate
  Quaternion Multiplication -  compute error quaternion : aerolibutil/Quaternion Multiplication
  Trigonometric Function : Trigonometry  Operator=acos
  Trigonometric Function1 : Trigonometry  Operator=asin
  choose the shorter  rotation : Switch  Criteria=u2 > Threshold
  get qw : Selector  InputPortWidth=4  IndexOptions=Index vector (dialog)  Indices=1  OutputSizes=1
  get qw1 : Selector  InputPortWidth=4  IndexOptions=Index vector (dialog)  Indices=1  OutputSizes=1
  "get qx, qy, qz" : Selector  InputPortWidth=4  IndexOptions=Index vector (dialog)  Indices=2:4  OutputSizes=1
  "get theta, phi1" : Selector  InputPortWidth=3  IndexOptions=Index vector (dialog)  Indices=[2 1]  OutputSizes=1
  "theta, phi local" : Outport
  wires:
  AirframeBus/1 -> Bus Selector/1
  Bus Selector/1 -> Direction Cosine Matrix  to Quaternions/1  "<DCM_be>"
  q_c/1 -> Quaternion Multiplication -  compute error quaternion/2
  choose the shorter  rotation/1 -> get qw/1, "get qx, qy, qz"/1  "q_corr"
  get qw/1 -> Trigonometric Function/1
  Trigonometric Function/1 -> Gain/1
  Gain/1 -> "If alpha_corr approaches zero,  q_e approaches 1 and c goes to infinity.  In that case, just replace the computed  correction angles by zeros"/2  "alpha_corr"
  "get qx, qy, qz"/1 -> Trigonometric Function1/1
  Trigonometric Function1/1 -> "If alpha_corr approaches zero,  q_e approaches 1 and c goes to infinity.  In that case, just replace the computed  correction angles by zeros"/1
  Constant1/1 -> "If alpha_corr approaches zero,  q_e approaches 1 and c goes to infinity.  In that case, just replace the computed  correction angles by zeros"/3
  "If alpha_corr approaches zero,  q_e approaches 1 and c goes to infinity.  In that case, just replace the computed  correction angles by zeros"/1 -> "get theta, phi1"/1
  "get theta, phi1"/1 -> Gain1/1
  Quaternion Conjugate/1 -> Quaternion Multiplication -  compute error quaternion/1
  Gain1/1 -> "theta, phi local"/1  "theta_local, phi_local"
  Quaternion Multiplication -  compute error quaternion/1 -> choose the shorter  rotation/3, Gain2/1  "q_corr"
  Gain2/1 -> choose the shorter  rotation/1, get qw1/1
  get qw1/1 -> choose the shorter  rotation/2
  Direction Cosine Matrix  to Quaternions/1 -> Quaternion Conjugate/1

== system Cularis_server_vortextest/Closed loop Cularis UAS, ID#2/Controllers/Attitude laws/Local rotation angle attitude  control/LQR pitch ==
  q : Inport
  theta : Inport  Port=2
  theta_c : Inport  Port=3
  Add1 : Sum  Inputs=-+
  Integrator1 : Integrator
  Mux2 : Mux  Inputs=3
  lquadr gain : Gain  Gain=uavsim.ap.control.lquadr.pitch.K  Multiplication=Matrix(K*u)
  de : Outport
  wires:
  q/1 -> Mux2/2
  Add1/1 -> Mux2/1, Integrator1/1  "e"
  theta_c/1 -> Add1/1
  theta/1 -> Add1/2
  Mux2/1 -> lquadr gain/1
  Integrator1/1 -> Mux2/3
  lquadr gain/1 -> de/1  "de"

== system Cularis_server_vortextest/Closed loop Cularis UAS, ID#2/Controllers/Attitude laws/Local rotation angle attitude  control/LQR roll ==
  phi : Inport
  phi_c : Inport  Port=2
  p : Inport  Port=3
  r : Inport  Port=4
  Add1 : Sum  Inputs=-+
  Demux : Demux  Outputs=2
  Integrator : Integrator
  Mux2 : Mux
  lquadr gain : Gain  Gain=uavsim.ap.control.lquadr.minimal.K  Multiplication=Matrix(K*u)
  da : Outport
  dr : Outport  Port=2
  wires:
  p/1 -> Mux2/2
  Demux/1 -> da/1
  Add1/1 -> Mux2/1, Integrator/1  "e"
  phi_c/1 -> Add1/1
  phi/1 -> Add1/2
  Mux2/1 -> lquadr gain/1
  Integrator/1 -> Mux2/4
  r/1 -> Mux2/3
  lquadr gain/1 -> Demux/1
  Demux/2 -> dr/1

== matlab function Closed loop Cularis UAS, ID#2/Controllers/Subsystem/Compute differential positions and velocities ==
  data: dx output Bus: Dx; closedloopmask_ID parameter double; VortexSig data_store_memory double
function dx = fcn(closedloopmask_ID)
%#codegen
global VortexSig;

dx = struct('dp_NED_m', zeros(10,3), 'dv_NED_mps', zeros(10,3));

for k=1:10
   dx.dp_NED_m(k, :) = VortexSig(k).p_NED_m - VortexSig(closedloopmask_ID).p_NED_m;
   dx.dv_NED_mps(k, :) = VortexSig(k).v_NED_mps - VortexSig(closedloopmask_ID).v_NED_mps;
end

end

== matlab function Virtual Leader, ID#1/Formation trajectory/MATLAB Function ==
  data: p_NED input double; v_NED input double; DCM_eg output double; c_NED input double; dp_g input double; p_c_NED output double
% Compute the DCM between the formation guidance frame (g) and the NED
% frame (e) for each UAS from the trajectory velocity and curvature vectors
% and the separation vectors between UAS.
function [DCM_eg, p_c_NED] = computeDCM_eg(p_NED,v_NED, c_NED, dp_g)
%#codegen
persistent last_uz;
if isempty(last_uz)
    last_uz = repmat([0 0 -1]', 1, 10);
end
p_c_NED = zeros(3,10);

% Compute the centripetal acceleration of the virtual leader:
% radius of the leader's instantaneous orbit:
a_centrip = zeros(3,1);
omega_vl = [0 0 0]';
if norm(c_NED) > eps
    r_vl = 1/(norm(c_NED));
    ur = -fflib_normalize(c_NED);
    omega_vl = cross(r_vl*ur, v_NED)/(r_vl^2);
    a_centrip = norm(omega_vl)^2 * r_vl*ur;
    bp = 0;
end

ux = fflib_normalize(v_NED);
[uz, last_uz] = compute_uz(ux, a_centrip, last_uz);

uy = cross(uz, ux);
DCM_eg = zeros(3,3,10);
DCM_eg(:, :, 1) = [ux uy uz];

% compute DCMs for remaining UASs's:
pddot_pre = a_centrip;
pdot_pre = v_NED;
omega_pre = omega_vl;
p_c_NED(:, 1) = p_NED;
for k=1:size(dp_g, 2)-1
    dp_e = DCM_eg(:, :, k) * dp_g(:, k);
    p_c_NED(:, k+1) = p_c_NED(:, k) + dp_e;
    pdot_fol = pdot_pre + cross(omega_pre, dp_e);
    pddot_fol = pddot_pre + cross(omega_pre, cross(omega_pre, dp_e));
    omega_fol_norm = (norm(pddot_fol)/norm(dp_e))^(1/2);
    omega_fol = omega_fol_norm * fflib_normalize(cross(pddot_fol, pdot_fol));
    if ~isempty(find(isnan(norm(omega_fol)), 1))
        omega_fol = zeros(3,1);
    end
    ux = fflib_normalize(pdot_fol);
    [uz, last_uz] = compute_uz(ux, pddot_fol, last_uz);
    uy = cross(uz, ux);
    DCM_eg(:, :, k+1) = [ux uy uz];
    pddot_pre = pddot_fol;
    pdot_pre = pdot_fol;
    omega_pre = omega_fol;
    bp = 0;
end
bp = 0;
end

function [uz, last_uz] = compute_uz(ux, a_centrip, lastuz_in)
last_uz = lastuz_in;
a_total = [0 0 9.81]' + a_centrip;
% Compute acceleration vector projected on y-z plane of the g frame:
a_total_yz = ffb_projectVectorOnPlane(a_total, ux);
% Total force defines z axis:
if norm(a_total_yz) > eps
    uz = fflib_normalize(a_total_yz);
    last_uz(:, 1) = uz;
else
    uz = lastuz_in(:, 1);
end
if uz(3) < 0
    bp = 0;
    uz = -uz;
end

end

== matlab function Closed loop Cularis UAS, ID#2/Controllers/Compute error measures/Compute differential positions and velocities ==
  data: dx output Bus: Dx; closedloopmask_ID parameter double; VortexSig data_store_memory double; dt output double
function [dx, dt] = fcn(closedloopmask_ID)
%#codegen
global VortexSig;

dx = struct('dp_NED_m', zeros(10,3), 'dv_NED_mps', zeros(10,3));
dt = zeros(10,1);
for k=1:10
   dx.dp_NED_m(k, :) = VortexSig(k).p_NED_m - VortexSig(closedloopmask_ID).p_NED_m;
   dx.dv_NED_mps(k, :) = VortexSig(k).v_NED_mps - VortexSig(closedloopmask_ID).v_NED_mps;
   dt(k, :) = VortexSig(k).timeOfLastUpdate - VortexSig(closedloopmask_ID).timeOfLastUpdate;   
end

end
